simulink library "INT_InjCrv_PiI1Cor"  (R2016b)
settings: Solver=VariableStepAuto  StartTime=0.0  StopTime=10.0  RelTol=1e-3
settings Model: Creator=mayongchao  LastModifiedBy=mayongchao

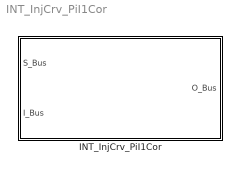
== system INT_InjCrv_PiI1Cor ==
  INT_InjCrv_PiI1Cor : Subsystem

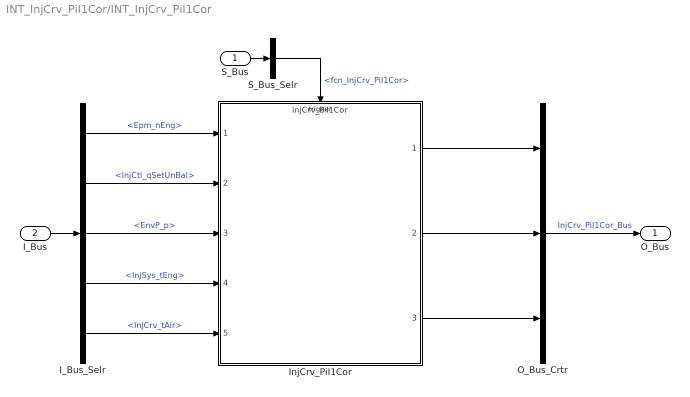
== system INT_InjCrv_PiI1Cor/INT_InjCrv_PiI1Cor ==
  S_Bus : Inport
  I_Bus : Inport  Port=2
  I_Bus_Selr : BusSelector  OutputSignals=Epm_nEng,InjCtl_qSetUnBal,EnvP_p,InjSys_tEng,InjCrv_tAir
  InjCrv_PiI1Cor : ModelReference  ModelNameDialog=InjCrv_PiI1Cor  SimulationMode=Normal  ModelReferenceVersion=1.37  TriggerPortName=function  TriggerPortTriggerType=function-call  TriggerPortStatesWhenEnabling=held
  O_Bus_Crtr : BusCreator  Inputs=3
  S_Bus_Selr : BusSelector  OutputSignals=fcn_InjCrv_PiI1Cor
  O_Bus : Outport
  wires:
  S_Bus_Selr/1 -> InjCrv_PiI1Cor/Trigger  "<fcn_InjCrv_PiI1Cor>"
  S_Bus/1 -> S_Bus_Selr/1
  I_Bus/1 -> I_Bus_Selr/1
  I_Bus_Selr/1 -> InjCrv_PiI1Cor/1  "<Epm_nEng>"
  I_Bus_Selr/2 -> InjCrv_PiI1Cor/2  "<InjCtl_qSetUnBal>"
  I_Bus_Selr/3 -> InjCrv_PiI1Cor/3  "<EnvP_p>"
  I_Bus_Selr/4 -> InjCrv_PiI1Cor/4  "<InjSys_tEng>"
  I_Bus_Selr/5 -> InjCrv_PiI1Cor/5  "<InjCrv_tAir>"
  O_Bus_Crtr/1 -> O_Bus/1  "InjCrv_PiI1Cor_Bus"
  InjCrv_PiI1Cor/1 -> O_Bus_Crtr/1
  InjCrv_PiI1Cor/2 -> O_Bus_Crtr/2
  InjCrv_PiI1Cor/3 -> O_Bus_Crtr/3
